simulink model "HVModAL_Fahrzeugmodell"  (R2015b)
settings: Solver=ode1  StartTime=0  StopTime=drp.driving_cycle.tstop  FixedStep=sim_params.Ts  RelTol=1e-5
PreLoadFcn:
  | % Add paths
  | addpath data
  | addpath(genpath('library'))
StartFcn:
  | Simulation.StartTime = tic;
StopFcn:
  | Simulation.DurationTime = toc(Simulation.StartTime);
undefined symbols (not defined in the file or in its folder): Batteries, BMS, BMS_Bat_, C_Nenn_DCDC1, C_Nenn_DCDC2, d2d, DC, DCDC_Converter_efficiency, DcDc_Converters, Dcl, drp, drv, elm, gen, gin, Hdc, hdc, HV, hvb, Hvb, ice, ldc, lib_dcl, lib_hdc, lib_hvb, lib_veh, Link, lossestable, mask_LUT_OCV, mask_LUT_OCV_SOC, mask_LUT_OCV_Temperature, mask_LUT_R, mask_LUT_Rs, mask_LUT_Rs_SOC, mask_LUT_Rs_Temperature, sim_params, speedvec, torquevec, tri, veh, Veh, Vehicle_Chassis
libraries: simulink x29, lib_tri_modules x7, lib_hdc_module x5, lib_gearbox x4, lib_hvb_battery_pack x3, cstblocks x3, PowerLimitBlock x2, MultiCellLibrary x2, lib_aux x1, lib_drv x1, lib_gen x1, lib_elm x1
(part 4 of 7)

== system HVModAL_Fahrzeugmodell/Traction Inverters (Tri)/Tri1/Thermal Model ==
  note: set enable equal 1 for Foster model
      | set enable equal 0 for junction model
  Plosses : Inport
  at_Ambient : Inport  Port=2
  Constant : Constant  Commented=on  Value=0
  Conventional thermal model : Subsystem  Commented=on
  Enable : Constant  Value=0
  Foster Model : Subsystem
  Logical Operator : Logic  Operator=NOT  Inputs=1  AllPortsSameDT=off  OutDataTypeStr=boolean
  Switch : Switch  Criteria=u2 ~= 0  ZeroCross=off
  Thermal Junction Model : Subsystem
  at_Junction_tri_vec : Outport
  wires:
  Foster Model/1(T_junction) -> Switch/1
  Constant/1 -> Conventional thermal model/Enable
  Thermal Junction Model/1(T_junction) -> Switch/3
  at_Ambient/1 -> Thermal Junction Model/2(T_amb), Foster Model/2(T_amb)
  Plosses/1 -> Thermal Junction Model/1(P_loss_vec), Foster Model/1(P_loss_vec)
  Enable/1 -> Logical Operator/1, Switch/2, Foster Model/Enable
  Switch/1 -> at_Junction_tri_vec/1
  Logical Operator/1 -> Thermal Junction Model/Enable

== system HVModAL_Fahrzeugmodell/Traction Inverters (Tri)/Tri1/Thermal Model old ==
  Plosses : Inport
  at_Ambient : Inport  Port=2
  Scope : Scope
  TJunc : Constant  Value=125
  Thermal Junction Model : Subsystem
  at_Junction : Outport
  wires:
  TJunc/1 -> at_Junction/1
  at_Ambient/1 -> Thermal Junction Model/2(T_amb)
  Plosses/1 -> Thermal Junction Model/1(P_loss_vec)
  Thermal Junction Model/1(T_junction) -> Scope/1

== system HVModAL_Fahrzeugmodell/Traction Inverters (Tri)/Tri1/mean_at_junction ==
  at_junction_tri_vec : Inport
  Constant : Constant  Value=12
  Divide : Product  Inputs=*/
  Sum of Elements : Sum  Inputs=+
  at_junction : Outport
  wires:
  at_junction_tri_vec/1 -> Sum of Elements/1
  Sum of Elements/1 -> Divide/1
  Constant/1 -> Divide/2
  Divide/1 -> at_junction/1

== system HVModAL_Fahrzeugmodell/Vehicle_Chassis (Veh)/Driving Data/Calculate Actual Speed ==
  m_red [kg] : Inport
  F_drive [N] : Inport  Port=2
  Integrator : Integrator
  Product : Product  Inputs=/*  SaturateOnIntegerOverflow=on  InputSameDT=on  OutDataTypeStr=Inherit: Same as first input
  v_actual [m/s] : Outport
  a_actual [m/s] : Outport  Port=2
  wires:
  Product/1 -> Integrator/1, a_actual [m/s]/1  "a_actual [m/s²]"
  Integrator/1 -> v_actual [m/s]/1  "v_actual [m/s]"
  m_red [kg]/1 -> Product/1
  F_drive [N]/1 -> Product/2

== system HVModAL_Fahrzeugmodell/Vehicle_Chassis (Veh)/Driving Data/Conversions ==
  v_actual (m/s) : Inport
  Emg_gearbox_vec : Inport  Port=2
  1/r_dyn : Gain  Gain=1/veh.wheel.radius  SaturateOnIntegerOverflow=on  OutDataTypeStr=Inherit: Same as input  ParamDataTypeStr=Inherit: Same as input
  Bus Selector : BusSelector  OutputSignals=BM on/off,gearboxratio_vec
  Demux : Demux
  Divide{,1..3} (4 alike) : Product  Inputs=*/
  Gain : Gain  Gain=veh.topology.boost_clutch
  Gain1 : Gain  Gain=veh.gearbox.gearbox2.ratio*elm.elm2.phys_avail  SaturateOnIntegerOverflow=on  OutDataTypeStr=Inherit: Same as input  ParamDataTypeStr=Inherit: Same as input
  Gain2 : Gain  Gain=veh.gearbox.gearbox1.ratio*elm.elm1.phys_avail  SaturateOnIntegerOverflow=on  OutDataTypeStr=Inherit: Same as input  ParamDataTypeStr=Inherit: Same as input
  Gain3 : Gain  Gain=veh.gearbox.gearbox3.ratio*elm.elm3.phys_avail  SaturateOnIntegerOverflow=on  OutDataTypeStr=Inherit: Same as input  ParamDataTypeStr=Inherit: Same as input
  Gain4 : Gain  Gain=veh.gearbox.gearbox4.ratio*elm.elm4.phys_avail  SaturateOnIntegerOverflow=on  OutDataTypeStr=Inherit: Same as input  ParamDataTypeStr=Inherit: Same as input
  Logical Operator : Logic  Operator=NOT  AllPortsSameDT=off  OutDataTypeStr=boolean
  Logical Operator1 : Logic  Operator=NOT  AllPortsSameDT=off  OutDataTypeStr=boolean
  Logical Operator2 : Logic  Operator=NOT  AllPortsSameDT=off  OutDataTypeStr=boolean
  Mux : Mux
  Product : Product  Inputs=3
  Product1 : Product  Inputs=3
  Switch : Switch  Criteria=u2 > Threshold
  Switch1 : Switch  Criteria=u2 > Threshold
  Terminator : Terminator
  Terminator2 : Terminator
  Terminator3 : Terminator
  const : Constant  Value=0
  const1 : Constant  Value=0
  "m/s -> km/h" : Gain  Gain=3.6  SaturateOnIntegerOverflow=on  OutDataTypeStr=Inherit: Same as input  ParamDataTypeStr=Inherit: Same as input
  "m/s -> rpm" : Gain  Gain=30/(pi*veh.wheel.radius)  SaturateOnIntegerOverflow=on  OutDataTypeStr=Inherit: Same as input  ParamDataTypeStr=Inherit: Same as input
  veh.topology.boost : Constant  Value=veh.topology.boost
  veh.topology.loc_boost : Constant  Value=veh.topology.loc_boost
  veh_n_motor_vec : Outport
  wires:
  Gain4/1 -> Divide/1
  Divide1/1 -> Mux/3
  Mux/1 -> veh_n_motor_vec/1
  "m/s -> km/h"/1 -> Terminator2/1  "v_actual (km/h)"
  1/r_dyn/1 -> Terminator/1  "n_wheels (rad/s)"
  "m/s -> rpm"/1 -> Terminator3/1, Gain2/1, Gain1/1, Gain3/1, Gain4/1  "n_wheels (rpm)"
  Divide3/1 -> Mux/1
  v_actual (m/s)/1 -> "m/s -> rpm"/1, 1/r_dyn/1, "m/s -> km/h"/1
  Emg_gearbox_vec/1 -> Bus Selector/1
  veh.topology.boost/1 -> Gain/1
  veh.topology.loc_boost/1 -> Logical Operator2/1, Product/3
  Bus Selector/1 -> Logical Operator1/1, Logical Operator/1  "<BM on/off>"
  Divide/1 -> Switch/3
  Product/1 -> Switch/2
  const/1 -> Switch/1
  Logical Operator/1 -> Product/1
  Gain/1 -> Product/2, Product1/2
  Product1/1 -> Switch1/2
  const1/1 -> Switch1/1
  Logical Operator1/1 -> Product1/1
  Switch1/1 -> Mux/2
  Divide2/1 -> Switch1/3
  Logical Operator2/1 -> Product1/3
  Switch/1 -> Mux/4
  Bus Selector/2 -> Demux/1  "<gearboxratio_vec>"
  Demux/4 -> Divide/2
  Gain3/1 -> Divide1/1
  Gain1/1 -> Divide2/1
  Demux/3 -> Divide1/2
  Demux/2 -> Divide2/2
  Gain2/1 -> Divide3/1
  Demux/1 -> Divide3/2

== system HVModAL_Fahrzeugmodell/Vehicle_Chassis (Veh)/Driving Forces/Aerodynamic Resistance ==
  v_desired [m/s] : Inport
  0.5*f_drag*A_front : Gain  Gain=veh.drag_coefficient*veh.front_area*0.5  SaturateOnIntegerOverflow=on  OutDataTypeStr=Inherit: Same as input  ParamDataTypeStr=Inherit: Same as input
  Air density : Gain  Gain=drp.airdensity  SaturateOnIntegerOverflow=on  OutDataTypeStr=Inherit: Same as input  ParamDataTypeStr=Inherit: Same as input
  Math Function : Math  Operator=square  SaturateOnIntegerOverflow=on
  F_aero [N] : Outport
  wires:
  0.5*f_drag*A_front/1 -> Air density/1
  v_desired [m/s]/1 -> Math Function/1
  Math Function/1 -> 0.5*f_drag*A_front/1
  Air density/1 -> F_aero [N]/1

== system HVModAL_Fahrzeugmodell/Vehicle_Chassis (Veh)/Driving Forces/Climbing Resistance ==
  gradient : Inport
  m_total * 9.81 : Gain  Gain=veh.totalweight*9.81  SaturateOnIntegerOverflow=on  OutDataTypeStr=Inherit: Same as input  ParamDataTypeStr=Inherit: Same as input
  sin(grad) : Trigonometry
  F_climb [N] : Outport
  wires:
  m_total * 9.81/1 -> F_climb [N]/1
  sin(grad)/1 -> m_total * 9.81/1
  gradient/1 -> sin(grad)/1

== system HVModAL_Fahrzeugmodell/Vehicle_Chassis (Veh)/Driving Forces/Rolling Resistance ==
  v_actual(m/s) : Inport
  gradient : Inport  Port=2
  9.81*m_total*f_roll : Gain  Gain=(veh.totalweight)*9.81*veh.wheel.rolling_resistance  SaturateOnIntegerOverflow=on  OutDataTypeStr=Inherit: Same as input  ParamDataTypeStr=Inherit: Same as input
  Constant : Constant  Value=0
  Product : Product
  Sign : Signum
  Switch : Switch  Threshold=0.1
  cos(grad) : Trigonometry  Operator=cos
  F_roll [N] : Outport
  wires:
  9.81*m_total*f_roll/1 -> Product/1
  gradient/1 -> cos(grad)/1
  cos(grad)/1 -> 9.81*m_total*f_roll/1
  Sign/1 -> Product/2
  Product/1 -> F_roll [N]/1
  v_actual(m/s)/1 -> Switch/1, Switch/2
  Constant/1 -> Switch/3
  Switch/1 -> Sign/1

== system HVModAL_Fahrzeugmodell/Vehicle_Chassis (Veh)/Wheel Model/  ==
  note: Wenn F_H > Fx : 1
  note: Abstand zwischen zwei Profilteilchen
  note: Länge eines Profilteilchens
  "F_x[N] " : Inport
  wheelLoad[N] : Inport  Port=2
  Abs : Abs
  Compare To Zero : simulink/Logic and Bit Operations/Compare To Zero  relop=>=  OutDataTypeStr=boolean
  Constant : Constant  Value=4
  Constant1 : Constant  Value=false
  Data Store Memory : DataStoreMemory  DataStoreName=Slip  ReadBeforeWriteMsg=warning  WriteAfterWriteMsg=warning  WriteAfterReadMsg=warning  InitialValue=false  ShowAdditionalParam=off  OutDataTypeStr=boolean
  Data Store Read : DataStoreRead  DataStoreName=Slip
  Gain : Gain  Gain=2
  Gain1 : Gain  Gain=2
  Gain2 : Gain  Gain=veh.wheel.coefficient_of_friction
  If : If  IfExpression=u1 <= 2000
  If Action Subsystem : Subsystem  TreatAsAtomicUnit=on
  Product : Product  Inputs=*/**///
  Product1 : Product  Inputs=*///
  Product2 : Product  Inputs=3
  Sqrt : Sqrt  SaturateOnIntegerOverflow=on
  Sum : Sum  Inputs=|++
  Sum1 : Sum  Inputs=+-
  Switch : Switch  Criteria=u2 > Threshold
  WheelRadius[m] : Constant  Value=veh.wheel.radius
  circumferentialTireRigidity[N/m] : Constant  Value=veh.wheel.c_t_rigidity
  distanceTireTread[m] : Constant  Value=veh.wheel.tread_distance
  lengthTireTread[m] : Constant  Value=veh.wheel.tread_length
  radialTireRigidity[N/m] : Constant  Value=veh.wheel.r_t_rigidity
  wheelspin : Outport
  Slip? : Outport  Port=2
  wires:
  Sum/1 -> Gain/1, Product/3
  lengthTireTread[m]/1 -> Sum/1
  distanceTireTread[m]/1 -> Sum/2
  "F_x[N] "/1 -> Product/1, Product2/3
  WheelRadius[m]/1 -> Product/2, Product1/2
  radialTireRigidity[N/m]/1 -> Product1/1, Product/4
  circumferentialTireRigidity[N/m]/1 -> Product/5
  wheelLoad[N]/1 -> Product1/3, Gain2/1, Product/6
  Constant/1 -> Product/7, Gain1/1
  Product/1 -> wheelspin/1
  Gain1/1 -> Product1/4
  Product1/1 -> Sqrt/1
  Sqrt/1 -> Product2/1
  Gain/1 -> Product2/2
  Gain2/1 -> Sum1/1
  Product2/1 -> Abs/1
  Abs/1 -> Sum1/2
  Data Store Read/1 -> Switch/2
  Switch/1 -> Slip?/1
  Constant1/1 -> Switch/3
  Compare To Zero/1 -> Switch/1
  Sum1/1 -> If/1, Compare To Zero/1
  If/1 -> If Action Subsystem/Action

== system HVModAL_Fahrzeugmodell/Vehicle_Chassis (Veh)/Wheel Model/F_x_wheelspin[N] ==
  F_wheel [N] : Inport
  angularVelocity [rad/s] : Inport  Port=2
  wheelload : Inport  Port=3
  Discrete Derivative : simulink/Discrete/Discrete Derivative  gainval=1  ICPrevScaledInput=0.0  InputProcessing=Inherited  OutMin=[]  OutMax=[]  OutDataType=fixdt(1, 16)  OutScaling=2^-10  DoSatur=off
  Gain : Gain  Gain=veh.wheel.coefficient_of_friction
  MinMax : MinMax  Inputs=2
  Product : Product  Inputs=*/
  Sum : Sum  Inputs=|+-
  r_dyn : Constant  Value=veh.wheel.radius
  "wheel_inertia " : Gain  Gain=veh.wheel.inertia
  F_x [N/m] : Outport
  wires:
  angularVelocity [rad/s]/1 -> Discrete Derivative/1
  r_dyn/1 -> Product/2
  F_wheel [N]/1 -> Sum/1
  Product/1 -> Sum/2
  Sum/1 -> MinMax/1
  MinMax/1 -> F_x [N/m]/1
  wheelload/1 -> Gain/1
  Gain/1 -> MinMax/2
  Discrete Derivative/1 -> "wheel_inertia "/1
  "wheel_inertia "/1 -> Product/1

== system HVModAL_Fahrzeugmodell/Vehicle_Chassis (Veh)/Wheel Model/Subsystem ==
  v_wheel [m/s] : Inport
  v/r : Gain  Gain=1/veh.wheel.radius
  angularVelocity[rad/s] : Outport
  wires:
  v_wheel [m/s]/1 -> v/r/1
  v/r/1 -> angularVelocity[rad/s]/1

== system HVModAL_Fahrzeugmodell/Vehicle_Chassis (Veh)/Wheel Model/wheelspin ==
  angularVelocity[rad/s] : Inport
  "wheelspin " : Inport  Port=2
  a_actual [m/s^2] : Inport  Port=3
  Slip? : Inport  Port=4
  v_wheel : Inport  Port=5
  Constant : Constant
  Constant1 : Constant
  Product : Product
  Product1 : Product  Inputs=*/
  Product2 : Product
  Sum : Sum  Inputs=|++  SaturateOnIntegerOverflow=on
  Sum1 : Sum  Inputs=|+-
  Switch : Switch  Criteria=u2 > Threshold
  Switch1 : Switch  Criteria=u2 ~= 0
  Switch2 : Switch  Criteria=u2 > Threshold
  rdyn : Constant  Value=veh.wheel.radius
  v_actual [m/s] : Outport
  wires:
  rdyn/1 -> Product/1
  angularVelocity[rad/s]/1 -> Product/2
  a_actual [m/s^2]/1 -> Switch/2
  Constant/1 -> Switch1/3, Sum/2
  Product/1 -> Product1/1, Product2/1
  Product1/1 -> Switch/3
  Sum1/1 -> Product2/2
  Product2/1 -> Switch/1
  Constant1/1 -> Sum1/1
  "wheelspin "/1 -> Sum1/2, Sum/1
  Sum/1 -> Switch1/2, Switch1/1
  Switch1/1 -> Product1/2
  Slip?/1 -> Switch2/2
  Switch/1 -> Switch2/1
  v_wheel/1 -> Switch2/3
  Switch2/1 -> v_actual [m/s]/1

== system HVModAL_Fahrzeugmodell/Visualization (Vis)/Subsystem1/Auxillaries (aux) ==
  Bus Selector : BusSelector  OutputSignals=Aux_P_lv_bat,Aux_P_dcLink
  Aux_P_lv_bat : Outport
  Aux_P_dcLink : Outport  Port=2
  wires:
  [Aux_BusPB_ToLogging] -> Bus Selector/1
  Bus Selector/1 -> Aux_P_lv_bat/1  "<Aux_P_lv_bat>"
  Bus Selector/2 -> Aux_P_dcLink/1  "<Aux_P_dcLink>"

== system HVModAL_Fahrzeugmodell/Visualization (Vis)/Subsystem1/DC-Link (Dcl) ==
  Bus Selector2 : BusSelector  OutputSignals=Dcl_U,Dcl_P_total,Dcl_P_totalwoHdcPdcLink,Hdc_P_dcLink
  Dcl_U : Outport
  Dcl_P_total : Outport  Port=2
  Dcl_P_totalwoHdcPdc : Outport  Port=3
  Hdc_P_dcLink : Outport  Port=4
  wires:
  [Dcl_BusPB_toworkspace] -> Bus Selector2/1
  Bus Selector2/1 -> Dcl_U/1  "<Dcl_U>"
  Bus Selector2/2 -> Dcl_P_total/1  "<Dcl_P_total>"
  Bus Selector2/3 -> Dcl_P_totalwoHdcPdc/1  "<Dcl_P_totalwoHdcPdcLink>"
  Bus Selector2/4 -> Hdc_P_dcLink/1  "<Hdc_P_dcLink>"

== system HVModAL_Fahrzeugmodell/Visualization (Vis)/Subsystem1/DC//DC Converter (hdc) ==
  Bus Selector : BusSelector  OutputSignals=Hdc_P_bat_vec,Hdc_P_dcLink_vec,Hdc_fac_eta_vec,Hdc_P_losses_vec
  Bus Selector1 : BusSelector  OutputSignals=Hdc_flg_error_vec,Hdc_P_max_vec,Hdc_at_Junction_vec
  Hdc_P_bat_vec : Outport
  Hdc_P_dclink_vec : Outport  Port=2
  Hdc_P_losses_vec : Outport  Port=3
  Hdc_fac_eta_vec : Outport  Port=4
  Hdc_error_vec : Outport  Port=5
  Hdc_Pmax_vec : Outport  Port=6
  Hdc_at_Junction_vec : Outport  Port=7
  wires:
  [Hdc_PBBus_toWorkspace] -> Bus Selector/1
  [Hdc_SWBus_toWorkspace] -> Bus Selector1/1
  Bus Selector/1 -> Hdc_P_bat_vec/1  "<Hdc_P_bat_vec>"
  Bus Selector/2 -> Hdc_P_dclink_vec/1  "<Hdc_P_dcLink_vec>"
  Bus Selector/3 -> Hdc_fac_eta_vec/1  "<Hdc_fac_eta_vec>"
  Bus Selector/4 -> Hdc_P_losses_vec/1  "<Hdc_P_losses_vec>"
  Bus Selector1/1 -> Hdc_error_vec/1  "<Hdc_flg_error_vec>"
  Bus Selector1/3 -> Hdc_at_Junction_vec/1  "<Hdc_at_Junction_vec>"
  Bus Selector1/2 -> Hdc_Pmax_vec/1  "<Hdc_P_max_vec>"

== system HVModAL_Fahrzeugmodell/Visualization (Vis)/Subsystem1/Driver (Drv) ==
  Bus Selector : BusSelector  OutputSignals=Drv_fac_PedAc
  Bus Selector1 : BusSelector  OutputSignals=Emg_T_elDemand_vec,Emg_T_mechDemand
  Bus Selector2 : BusSelector  OutputSignals=Drp_v_vehDesired
  Gain1 : Gain  Gain=3.6
  Sum of Elements : Sum  Inputs=+
  fac_pedAcc : Outport
  Emg_T_el_demand : Outport  Port=2
  Emg_T_mech_demand : Outport  Port=3
  v_cycle(km/h) : Outport  Port=4
  wires:
  Bus Selector/1 -> fac_pedAcc/1  "<Drv_fac_PedAc>"
  [Drv_SWBus_toworkspace] -> Bus Selector/1
  [EMG_BusSW_ToLogging] -> Bus Selector1/1
  Bus Selector1/2 -> Emg_T_mech_demand/1  "<Emg_T_mechDemand>"
  Bus Selector1/1 -> Sum of Elements/1  "<Emg_T_elDemand_vec>"
  Sum of Elements/1 -> Emg_T_el_demand/1
  Gain1/1 -> v_cycle(km/h)/1  "v_cycle(km/h)"
  [Drp_SWBus_toworkspace] -> Bus Selector2/1
  Bus Selector2/1 -> Gain1/1  "<Drp_v_vehDesired>"

== system HVModAL_Fahrzeugmodell/Visualization (Vis)/Subsystem1/EMS ==
  Bus Selector : BusSelector  OutputSignals=Emg_fac_powerDistribution_vec,Emg_T_elDemand_vec,Emg_Degradation_vec
  Demux : Demux  Commented=on  Outputs=5
  Demux1 : Demux
  Emg_fac_powerDristri_Bat1 : Outport
  Emg_fac_powerDristri_Bat2 : Outport  Port=2
  Emg_fac_powerDristri_Bat3 : Outport  Port=3
  Emg_fac_powerDristri_Bat4 : Outport  Port=4
  Emg_fac_powerDristri_Bat5 : Outport  Port=5
  Emg_T_elDemand_Inv1 : Outport  Port=6
  Emg_T_elDemand_Inv2 : Outport  Port=7
  Emg_Degradation : Outport  Port=8
  wires:
  Demux/1 -> Emg_fac_powerDristri_Bat1/1
  Demux/2 -> Emg_fac_powerDristri_Bat2/1
  Demux/3 -> Emg_fac_powerDristri_Bat3/1
  Demux/4 -> Emg_fac_powerDristri_Bat4/1
  Demux/5 -> Emg_fac_powerDristri_Bat5/1
  Demux1/1 -> Emg_T_elDemand_Inv1/1
  Demux1/2 -> Emg_T_elDemand_Inv2/1
  [EMG_BusSW_ToLogging] -> Bus Selector/1
  Bus Selector/1 -> Demux/1  "<Emg_fac_powerDistribution_vec>"
  Bus Selector/2 -> Demux1/1  "<Emg_T_elDemand_vec>"
  Bus Selector/3 -> Emg_Degradation/1  "<Emg_Degradation_vec>"

== system HVModAL_Fahrzeugmodell/Visualization (Vis)/Subsystem1/Elm ==
  Bus Selector : BusSelector  OutputSignals=Elm_T_el_vec,Elm_I_abc_vec,Elm_P_TD_actual_vec
  Bus Selector1 : BusSelector  OutputSignals=Elm_P_losses_vec,Tri_Pmax_elm_vec,elm_at_endWindingsMagnet_vec
  Demux : Demux
  Elm_T_el_vec : Outport
  Elm_P_actual_vec : Outport  Port=2
  Elm_P_losses_vec : Outport  Port=3
  Elm1_I_abc : Outport  Port=4
  Elm_Pmax_vec : Outport  Port=5
  Elm_at_endWindingsMagnet_vec : Outport  Port=6
  wires:
  [Elm_BusPB_toworkspace] -> Bus Selector/1
  Bus Selector/1 -> Elm_T_el_vec/1  "<Elm_T_el_vec>"
  Bus Selector/2 -> Demux/1  "<Elm_I_abc_vec>"
  Demux/1 -> Elm1_I_abc/1  "Elm_I_abc"
  Bus Selector/3 -> Elm_P_actual_vec/1  "<Elm_P_TD_actual_vec>"
  [Tri_BusSW_toWorkspace] -> Bus Selector1/1
  Bus Selector1/1 -> Elm_P_losses_vec/1  "<Elm_P_losses_vec>"
  Bus Selector1/2 -> Elm_Pmax_vec/1  "<Tri_Pmax_elm_vec>"
  Bus Selector1/3 -> Elm_at_endWindingsMagnet_vec/1  "<elm_at_endWindingsMagnet_vec>"

== system HVModAL_Fahrzeugmodell/Visualization (Vis)/Subsystem1/HV-Batteries (hvb) ==
  Abs : Abs
  Add : Sum
  Bus Selector : BusSelector  OutputSignals=PB_Bat1,PB_Bat2
  Bus Selector1 : BusSelector  OutputSignals=Total_Voltage_V,Total_Current_A,SOC_Vector_Percent,Total_Dissipation_Power_W
  Bus Selector2 : BusSelector  OutputSignals=Total_Voltage_V,Total_Current_A,SOC_Vector_Percent
  Bus Selector3 : BusSelector  OutputSignals=SB_Bat1,SB_Bat2
  Bus Selector4 : BusSelector  OutputSignals=P_max_discharge_10s_W
  Bus Selector5 : BusSelector  OutputSignals=P_max_discharge_10s_W
  Constant : Constant  Value=0
  Display : Display
  Display1 : Display
  Display2 : Display
  Gain : Gain  Gain=1/3600
  Gain1 : Gain  Gain=1/3600
  Gain2 : Gain  Gain=1/3600
  Integrator : Integrator
  Integrator1 : Integrator
  Integrator2 : Integrator
  Product : Product
  Product1 : Product
  Switch : Switch  Criteria=u2 > Threshold
  Switch1 : Switch  Criteria=u2 > Threshold
  Hvb_Bat1_U : Outport
  Hvb_Bat1_I : Outport  Port=2
  Hvb_Bat1_P : Outport  Port=3
  Hvb_Bat1_SOC : Outport  Port=4
  Hvb_Bat2_U : Outport  Port=5
  Hvb_Bat2_I : Outport  Port=6
  Hvb_Bat2_P : Outport  Port=7
  Hvb_Bat2_SOC : Outport  Port=8
  Hvb_Bat1_P_max_disch : Outport  Port=9
  Hvb_Bat2_P_max_disch : Outport  Port=10
  Hvb_Bat_P_max_disch : Outport  Port=11
  Hvb_Bat1_Plosses : Outport  Port=12
  wires:
  [Hvb_PBbus_toworkspace] -> Bus Selector/1
  Bus Selector/1 -> Bus Selector1/1  "<PB_Bat1>"
  Bus Selector/2 -> Bus Selector2/1  "<PB_Bat2>"
  Bus Selector1/1 -> Product/1, Hvb_Bat1_U/1  "<Total_Voltage_V>"
  Bus Selector1/2 -> Product/2, Hvb_Bat1_I/1  "<Total_Current_A>"
  Bus Selector1/3 -> Hvb_Bat1_SOC/1  "<SOC_Vector_Percent>"
  Product/1 -> Switch/1, Switch1/3, Switch1/2, Switch/2, Abs/1, Hvb_Bat1_P/1  "Hvb_Bat1_P"
  Bus Selector2/1 -> Hvb_Bat2_U/1, Product1/1  "<Total_Voltage_V>"
  Bus Selector2/2 -> Product1/2, Hvb_Bat2_I/1  "<Total_Current_A>"
  Bus Selector2/3 -> Hvb_Bat2_SOC/1  "<SOC_Vector_Percent>"
  Product1/1 -> Hvb_Bat2_P/1  "Hvb_Bat2_P"
  [Hvb_SWbus_toworkspace] -> Bus Selector3/1
  Bus Selector3/1 -> Bus Selector4/1  "<SB_Bat1>"
  Bus Selector3/2 -> Bus Selector5/1  "<SB_Bat2>"
  Bus Selector4/1 -> Add/1, Hvb_Bat1_P_max_disch/1  "<P_max_discharge_10s_W>"
  Bus Selector5/1 -> Add/2, Hvb_Bat2_P_max_disch/1  "<P_max_discharge_10s_W>"
  Add/1 -> Hvb_Bat_P_max_disch/1
  Bus Selector1/4 -> Hvb_Bat1_Plosses/1  "<Total_Dissipation_Power_W>"
  Switch/1 -> Integrator/1
  Constant/1 -> Switch1/1, Switch/3
  Switch1/1 -> Integrator1/1
  Abs/1 -> Integrator2/1
  Integrator1/1 -> Gain1/1
  Integrator/1 -> Gain/1
  Integrator2/1 -> Gain2/1
  Gain2/1 -> Display/1
  Gain/1 -> Display2/1
  Gain1/1 -> Display1/1

== system HVModAL_Fahrzeugmodell/Visualization (Vis)/Subsystem1/LV-DCDC (ldc) ==
  Bus Selector1 : BusSelector  OutputSignals=Ldc_Pmax_vec,Ldc_atJunction_vec,Ldc_error_vec
  Bus Selector2 : BusSelector  OutputSignals=Ldc_P_LvBat,Ldc_P_HvBat_vec,Ldc_P_dcLink
  Ldc_P_Lv_bat : Outport
  Ldc_P_HvBat_vec : Outport  Port=2
  Ldc_P_dcLink : Outport  Port=3
  Ldc_atJunction_vec : Outport  Port=4
  Ldc_Pmax_vec : Outport  Port=5
  Ldc_error_vec : Outport  Port=6
  wires:
  [LDC_BusSB_ToLogging] -> Bus Selector1/1
  Bus Selector1/1 -> Ldc_Pmax_vec/1  "<Ldc_Pmax_vec>"
  Bus Selector1/2 -> Ldc_atJunction_vec/1  "<Ldc_atJunction_vec>"
  Bus Selector1/3 -> Ldc_error_vec/1  "<Ldc_error_vec>"
  [LDC_BusPB_ToLogging] -> Bus Selector2/1
  Bus Selector2/1 -> Ldc_P_Lv_bat/1  "<Ldc_P_LvBat>"
  Bus Selector2/2 -> Ldc_P_HvBat_vec/1  "<Ldc_P_HvBat_vec>"
  Bus Selector2/3 -> Ldc_P_dcLink/1  "<Ldc_P_dcLink>"

== system HVModAL_Fahrzeugmodell/Visualization (Vis)/Subsystem1/Subsystem1 ==
  Bus Selector1 : BusSelector  OutputSignals=Drp_v_vehDesired
  Bus Selector2 : BusSelector  OutputSignals=Veh_random
  Gain : Gain  Gain=3.6
  Gain1 : Gain  Gain=3.6
  Sum : Sum  Inputs=+-
  v_deviation(km/h) : Outport
  wires:
  Bus Selector1/1 -> Gain1/1  "<Drp_v_vehDesired>"
  Sum/1 -> v_deviation(km/h)/1  "v_deviation(km/h)"
  Gain/1 -> Sum/2  "v_actual(km/h)"
  [Drp_SWBus_toworkspace] -> Bus Selector1/1
  Bus Selector2/1 -> Gain/1  "<Veh_random>"
  [Veh_SWBus_toworkspace] -> Bus Selector2/1
  Gain1/1 -> Sum/1  "v_cycle(km/h)"

== system HVModAL_Fahrzeugmodell/Visualization (Vis)/Subsystem1/Traction Inverters(Tri) ==
  Bus Selector1 : BusSelector  OutputSignals=Tri_Pmax_vec,Tri_fac_eta,Tri_at_Junction_vec
  Bus Selector2 : BusSelector  OutputSignals=Tri_P_dcLink_vec,Tri_P_losses_vec
  Tri_P_dcLink : Outport
  Tri_P_losses : Outport  Port=2
  Tri_eta : Outport  Port=3
  Tri_Pmax : Outport  Port=4
  Tri_atJunction : Outport  Port=5
  wires:
  [Tri_BusPB_toWorkspace] -> Bus Selector2/1
  [Tri_BusSW_toWorkspace] -> Bus Selector1/1
  Bus Selector2/1 -> Tri_P_dcLink/1  "<Tri_P_dcLink_vec>"
  Bus Selector2/2 -> Tri_P_losses/1  "<Tri_P_losses_vec>"
  Bus Selector1/1 -> Tri_Pmax/1  "<Tri_Pmax_vec>"
  Bus Selector1/2 -> Tri_eta/1  "<Tri_fac_eta>"
  Bus Selector1/3 -> Tri_atJunction/1  "<Tri_at_Junction_vec>"

== system HVModAL_Fahrzeugmodell/Visualization (Vis)/Subsystem1/Vehicle (veh) ==
  Bus Selector2 : BusSelector  OutputSignals=Veh_DrivingForces_N,Veh_a_actual,Veh_random,Veh_v_actual,Veh_Ploss_gearbox_vec
  Demux : Demux  Outputs=5
  Sum : Sum  Inputs=+-|
  Sum of Elements : Sum  Inputs=+
  Veh_F_aero : Outport
  Veh_F_climb : Outport  Port=2
  Veh_F_drive : Outport  Port=3
  Veh_F_roll : Outport  Port=4
  Veh_F_acc : Outport  Port=5
  Veh_a_actual : Outport  Port=6
  Veh_v_actual : Outport  Port=7
  Veh_v_actual-v_wheel : Outport  Port=8
  Veh_Ploss_gearbox : Outport  Port=9
  wires:
  [Veh_SWBus_toworkspace] -> Bus Selector2/1
  Bus Selector2/1 -> Demux/1  "<Veh_DrivingForces_N>"
  Demux/1 -> Veh_F_acc/1
  Demux/2 -> Veh_F_aero/1
  Demux/3 -> Veh_F_climb/1
  Demux/4 -> Veh_F_drive/1
  Demux/5 -> Veh_F_roll/1
  Bus Selector2/2 -> Veh_a_actual/1  "<Veh_a_actual>"
  Bus Selector2/3 -> Sum/1, Veh_v_actual/1  "<Veh_random>"
  Bus Selector2/4 -> Sum/2  "<Veh_v_actual>"
  Sum/1 -> Veh_v_actual-v_wheel/1
  Bus Selector2/5 -> Sum of Elements/1  "<Veh_Ploss_gearbox_vec>"
  Sum of Elements/1 -> Veh_Ploss_gearbox/1

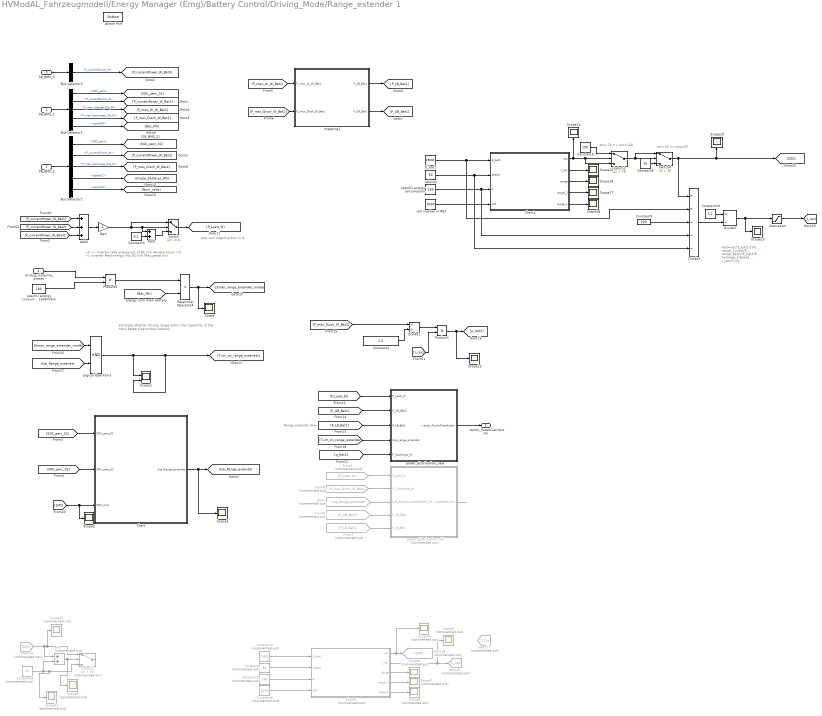
== system HVModAL_Fahrzeugmodell/Energy Manager (Emg)/Battery Control/Driving_Mode/Range_extender 1 ==
  note: pos. and negative
      | but != 0
  note: >0 --> Inverter take energy out of DC link (Acceleration)
      | <0 --> Inverter feed energy into DC link (Recuperation)
  note: Range extender 5kw
  note: estimate whether driving range within the capability of the main battery(secondary battery
  note: soc<30 => soc=30
  note: soc>79 => soc=100
  note: rest=soc*E_bat1/100;...
      |  range_1=rest/E;...
      | range_bat1=E_bat1/E;...
      |  t=range_1/speed;...
      |  I_rex=3.1/t;...
  SB_BMS_1 : Inport
  SB_BMS_2 : Inport  Port=2
  SB_BMS_3 : Inport  Port=3
  driving_distance_preset : Inport  Port=4
  Action Port : ActionPort
  Add : Sum  Commented=on
  Add1 : Sum
  Add2 : Sum  Inputs=+++
  Bus Selector1 : BusSelector  OutputSignals=SOC_perc,P_currentPower_W,P_max_charge_10s_W,P_max_discharge_10s_W,signal20
  Bus Selector2 : BusSelector  OutputSignals=SOC_perc,P_currentPower_W,P_max_discharge_10s_W,signal21,signal22
  Bus Selector3 : BusSelector  OutputSignals=P_currentPower_W
  Chart : Stateflow chart  TreatAsAtomicUnit=on
      settings: PermitHierarchicalResolution=ParametersOnly
  Chart1 : Stateflow chart  TreatAsAtomicUnit=on
      settings: PermitHierarchicalResolution=ParametersOnly
  Chart3 : Stateflow chart  Commented=on  TreatAsAtomicUnit=on
      settings: PermitHierarchicalResolution=ParametersOnly
  Constant : Constant  Commented=on  Value=50
  Constant1 : Constant  Commented=on  Value=25000
  Constant10 : Constant  Value=3.1
  Constant2 : Constant  Value=2.5
  Constant3 : Constant  Value=0.1
  Constant4 : Constant  Commented=on  Value=10
  Constant5 : Constant  Value=100
  Constant6 : Constant  Commented=on  Value=4200
  Constant7 : Constant  Commented=on  Value=160
  Constant8 : Constant  Value=30
  Constant9 : Constant  Value=100
  Divide1 : Product  Inputs=*/
  Divide2 : Product  Inputs=**///
  Divide3 : Product  Inputs=*/
  E_bat1 : Constant  Value=25000
  From : From  Commented=on  GotoTag=Use_Range_extender  TagVisibility=global
  From1 : From  Commented=on  GotoTag=P_Load_W
  From10 : From  Commented=on  GotoTag=SOC
  From7 : From  Commented=on  GotoTag=P_LB_Bat1
  From8 : From  Commented=on  GotoTag=P_UB_Bat1
  From9 : From  Commented=on  GotoTag=P_max_Disch_W_Bat2
  Gain : Gain  Gain=-1
  Goto17 : Goto  Commented=on  GotoTag=I_rex
  Goto18 : Goto  Commented=on  GotoTag=SOC
  Goto21 : Goto  Commented=on  GotoTag=I_rex
  Logical Operator3 : Logic  AllPortsSameDT=off  OutDataTypeStr=boolean
  Product1 : Product
  Product2 : Product
  Relational Operator4 : RelationalOperator  Operator=>  OutDataTypeStr=boolean
  Saturation : Saturate  UpperLimit=3  LowerLimit=0
  Scope{,2..3,12..19} (11 alike) : Scope
  Scope1 : Scope  NumInputPorts=2
  Scope{4..11} (8 alike) : Scope  Commented=on
  Switch : Switch  Criteria=u2 ~= 0  Threshold=0.5
  Switch1 : Switch  Commented=on  Criteria=u2 > Threshold  Threshold=20
  Switch2 : Switch  Criteria=u2 > Threshold  Threshold=79
  Switch4 : Switch  Criteria=u2 > Threshold  Threshold=30
  cell number in REX : Constant  Value=4000
  mapping1 : Subsystem  AncestorBlock=PowerDistribution_Dynamic_algo/Dynamic_power_distribution_1av_HE_AND_2av_HP/mapping1  TreatAsAtomicUnit=on
  power_distribution_new : Subsystem
  power_distribution_old : Subsystem  Commented=on
  specific energy consumption : Constant  Value=160
  specific energy consumption 160Wh/Km : Constant  Value=160
  velocity : Constant  Value=50
  vector_PowerDistribution : Outport
  tag scope: Use_Range_extender=global
  wires:
  Chart/1(Use_Range_extender) -> Scope3/1, [Use_Range_extender]
  Gain/1 -> Add1/1, Switch/2, Switch/1
  Constant3/1 -> Add1/2
  Add1/1 -> Switch/3
  [P_currentPower_W_Bat2] -> Add2/2
  [P_currentPower_W_Bat1] -> Add2/1
  Add2/1 -> Gain/1
  SB_BMS_1/1 -> Bus Selector1/1
  SB_BMS_2/1 -> Bus Selector2/1
  [SOC_perc_02] -> Chart/2(SOC_perc_02)
  [SOC_perc_01] -> Chart/1(SOC_perc_01)
  Bus Selector2/1 -> [SOC_perc_02]  "<SOC_perc>"
  Bus Selector2/2 -> [P_currentPower_W_Bat2]  "<P_currentPower_W>"
  Bus Selector1/2 -> [P_currentPower_W_Bat1]  "<P_currentPower_W>"
  Bus Selector1/1 -> [SOC_perc_01]  "<SOC_perc>"
  SB_BMS_3/1 -> Bus Selector3/1
  Bus Selector3/1 -> [P_currentPower_W_Bat3]  "<P_currentPower_W>"
  [P_currentPower_W_Bat3] -> Add2/3
  From1/1 -> power_distribution_old/1(P_Load_W)
  From9/1 -> power_distribution_old/2(P2_discharge_W)
  From/1 -> power_distribution_old/3(Use_Range_extender)
  Bus Selector1/3 -> [P_max_ch_W_Bat1]  "<P_max_charge_10s_W>"
  Bus Selector1/4 -> [P_max_Disch_W_Bat1]  "<P_max_discharge_10s_W>"
  [P_max_ch_W_Bat1] -> mapping1/1(P_max_ch_W_Bat1)
  [P_max_Disch_W_Bat1] -> mapping1/2(P_max_Disch_W_Bat1)
  mapping1/1(P_LB_Bat1) -> [P_LB_Bat1]
  mapping1/2(P_UB_Bat1) -> [P_UB_Bat1]
  From8/1 -> power_distribution_old/4(P_UB_Bat1)
  From7/1 -> power_distribution_old/5(P_LB_Bat1)
  Bus Selector2/3 -> [P_max_Disch_W_Bat2]  "<P_max_discharge_10s_W>"
  Switch/1 -> [P_Load_W]
  power_distribution_old/1(vector_PowerDistribution) -> ?
  Bus Selector1/5 -> [Bat_Wh]  "<signal20>"
  [Bat_Wh] -> Relational Operator4/2
  [P_Load_W] -> power_distribution_new/1(P_Load_W)
  [p_bat2] -> power_distribution_new/5(P_discharge_W)
  [P_LB_Bat1] -> power_distribution_new/3(P_LB_Bat1)
  [P_UB_Bat1] -> power_distribution_new/2(P_UB_Bat1)
  power_distribution_new/1(vector_PowerDistribution) -> vector_PowerDistribution/1
  Relational Operator4/1 -> Scope/1, [Enter_range_extender_mode]
  [Enter_range_extender_mode] -> Logical Operator3/1
  [Use_Range_extender] -> Logical Operator3/2
  [Turn_on_range_extender] -> power_distribution_new/4(Use_range_extender)
  Logical Operator3/1 -> Scope1/2, [Turn_on_range_extender], Scope1/1
  Product1/1 -> Scope12/1, [p_bat2]
  Constant2/1 -> Divide1/2
  [P_max_Disch_W_Bat2] -> Divide1/1
  Divide1/1 -> Product1/1
  Bus Selector2/4 -> [Single_battery2_Wh]  "<signal21>"
  Bus Selector2/5 -> [Num_cells]  "<signal22>"
  Constant/1 -> Chart3/2(speed)
  Constant7/1 -> Chart3/3(E)
  Chart3/2(I_rex) -> Goto21/1, Scope5/1
  Chart3/3(range) -> Scope6/1
  Chart3/1(soc) -> Goto18/1, Scope4/1
  Chart3/4(range_2) -> Scope7/1
  Chart3/5(range_1) -> Scope8/1
  From10/1 -> Add/1, Scope10/1, Switch1/1
  Constant4/1 -> Add/2, Scope11/1, Switch1/3
  Add/1 -> Scope9/1, Switch1/2
  [SOC] -> Chart/3(SOC_limit), Scope2/1
  Constant6/1 -> Chart3/4(cell)
  Constant1/1 -> Chart3/1(E_bat1)
  driving_distance_preset/1 -> Product2/1
  specific energy consumption 160Wh/Km/1 -> Product2/2
  Product2/1 -> Relational Operator4/1
  [I_rex] -> Product1/2
  Constant5/1 -> Switch2/1
  Switch2/1 -> Switch4/1, Switch4/2
  Constant8/1 -> Switch4/3
  Divide2/1 -> Divide3/2
  Switch4/1 -> [SOC], Scope19/1, Divide2/1
  Constant9/1 -> Divide2/3
  Divide3/1 -> Saturation/1, Scope13/1
  Constant10/1 -> Divide3/1
  velocity/1 -> Divide2/5, Chart1/2(speed)
  specific energy consumption/1 -> Divide2/4, Chart1/3(E)
  Chart1/2(I_rex) -> Scope15/1
  Chart1/1(soc) -> Scope14/1, Switch2/3, Switch2/2
  Chart1/3(range) -> Scope16/1
  Chart1/4(range_2) -> Scope17/1
  Chart1/5(range_1) -> Scope18/1
  cell number in REX/1 -> Chart1/4(cell)
  E_bat1/1 -> Divide2/2, Chart1/1(E_bat1)
  Saturation/1 -> [I_rex]

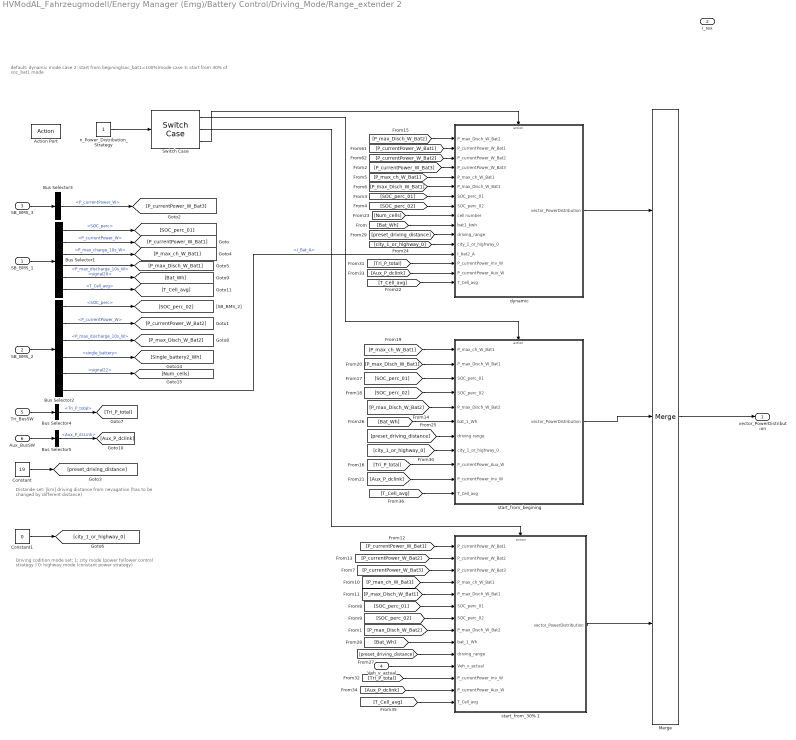
== system HVModAL_Fahrzeugmodell/Energy Manager (Emg)/Battery Control/Driving_Mode/Range_extender 2 ==
  note: default: dynamic mode
      | case 2: start from begining(soc_bat1=100%)mode
      | case 3: start from 30% of soc_bat1 mode
  note: Distande set: [km]
      | driving distance from nevagation
      | (has to be changed by different distance)
  note: Driving codition mode set:
      | 1: city mode (power follower control strategy )
      | 0: highway mode (constant power strategy)
  SB_BMS_1 : Inport
  SB_BMS_2 : Inport  Port=2
  SB_BMS_3 : Inport  Port=3
  Veh_v_actual : Inport  Port=4
  Tri_BusSW : Inport  Port=5
  "Aux_BusSW " : Inport  Port=6
  Action Port : ActionPort  ActionType=case
  Bus Selector1 : BusSelector  OutputSignals=SOC_perc,P_currentPower_W,P_max_charge_10s_W,P_max_discharge_10s_W,signal20,T_Cell_avg
  Bus Selector2 : BusSelector  OutputSignals=SOC_perc,P_currentPower_W,P_max_discharge_10s_W,single_battery,signal22,I_Bat_A
  Bus Selector3 : BusSelector  OutputSignals=P_currentPower_W
  Bus Selector4 : BusSelector  OutputSignals=Tri_P_total
  Bus Selector5 : BusSelector  OutputSignals=Aux_P_dcLink
  Constant : Constant  Value=19
  Constant1 : Constant  Value=0
  Merge : Merge  Inputs=3
  Switch Case : SwitchCase  CaseConditions={2, 3}
  dynamic : Subsystem
  n_Power_Distribution_Strategy : Constant
  start_from_30% 1 : Subsystem
  "start_from_begining " : Subsystem
  vector_PowerDistribution : Outport
  I_rex : Outport  Port=2
  wires:
  SB_BMS_1/1 -> Bus Selector1/1
  SB_BMS_2/1 -> Bus Selector2/1
  Bus Selector2/1 -> [SOC_perc_02]  "<SOC_perc>"
  Bus Selector2/2 -> [P_currentPower_W_Bat2]  "<P_currentPower_W>"
  Bus Selector1/2 -> [P_currentPower_W_Bat1]  "<P_currentPower_W>"
  Bus Selector1/1 -> [SOC_perc_01]  "<SOC_perc>"
  SB_BMS_3/1 -> Bus Selector3/1
  Bus Selector3/1 -> [P_currentPower_W_Bat3]  "<P_currentPower_W>"
  Bus Selector1/3 -> [P_max_ch_W_Bat1]  "<P_max_charge_10s_W>"
  Bus Selector1/4 -> [P_max_Disch_W_Bat1]  "<P_max_discharge_10s_W>"
  Bus Selector2/3 -> [P_max_Disch_W_Bat2]  "<P_max_discharge_10s_W>"
  Bus Selector1/5 -> [Bat_Wh]  "<signal20>"
  Bus Selector2/4 -> [Single_battery2_Wh]  "<single_battery>"
  Bus Selector2/5 -> [Num_cells]  "<signal22>"
  [P_max_Disch_W_Bat2] -> dynamic/1(P_max_Disch_W_Bat2)
  [P_currentPower_W_Bat1] -> dynamic/2(P_currentPower_W_Bat1)
  [P_currentPower_W_Bat2] -> dynamic/3(P_currentPower_W_Bat2)
  [P_currentPower_W_Bat3] -> dynamic/4(P_currentPower_W_Bat3)
  [P_max_ch_W_Bat1] -> dynamic/5(P_max_ch_W_Bat1)
  [P_max_Disch_W_Bat1] -> dynamic/6(P_max_Disch_W_Bat1)
  [SOC_perc_01] -> dynamic/7(SOC_perc_01)
  [SOC_perc_02] -> dynamic/8(SOC_perc_02)
  n_Power_Distribution_Strategy/1 -> Switch Case/1
  start_from_30% 1/1(vector_PowerDistribution) -> Merge/3
  [P_max_Disch_W_Bat2] -> "start_from_begining "/5(P_max_Disch_W_Bat2)
  [P_max_ch_W_Bat1] -> "start_from_begining "/1(P_max_ch_W_Bat1)
  [P_max_Disch_W_Bat1] -> "start_from_begining "/2(P_max_Disch_W_Bat1)
  [SOC_perc_01] -> "start_from_begining "/3(SOC_perc_01)
  [SOC_perc_02] -> "start_from_begining "/4(SOC_perc_02)
  Switch Case/3 -> dynamic/Action
  Switch Case/2 -> start_from_30% 1/Action
  Switch Case/1 -> "start_from_begining "/Action
  Merge/1 -> vector_PowerDistribution/1
  dynamic/1(vector_PowerDistribution) -> Merge/1
  Constant/1 -> [preset_driving_distance]
  [Bat_Wh] -> dynamic/10(bat1_kwh)
  [Num_cells] -> dynamic/9(cell number)
  [preset_driving_distance] -> dynamic/11(driving_range)
  [preset_driving_distance] -> "start_from_begining "/7(driving range)
  [Bat_Wh] -> "start_from_begining "/6(bat_1_Wh)
  [P_currentPower_W_Bat1] -> start_from_30% 1/1(P_currentPower_W_Bat1)
  [P_currentPower_W_Bat2] -> start_from_30% 1/2(P_currentPower_W_Bat2)
  [P_currentPower_W_Bat3] -> start_from_30% 1/3(P_currentPower_W_Bat3)
  [P_max_ch_W_Bat1] -> start_from_30% 1/4(P_max_ch_W_Bat1)
  [P_max_Disch_W_Bat1] -> start_from_30% 1/5(P_max_Disch_W_Bat1)
  [SOC_perc_01] -> start_from_30% 1/6(SOC_perc_01)
  [SOC_perc_02] -> start_from_30% 1/7(SOC_perc_02)
  [P_max_Disch_W_Bat2] -> start_from_30% 1/8(P_max_Disch_W_Bat2)
  [preset_driving_distance] -> start_from_30% 1/10(driving_range)
  [Bat_Wh] -> start_from_30% 1/9(bat_1_Wh)
  Constant1/1 -> [city_1_or_highway_0]
  "start_from_begining "/1(vector_PowerDistribution) -> Merge/2
  [city_1_or_highway_0] -> dynamic/12(city_1_or_highway_0)
  [city_1_or_highway_0] -> "start_from_begining "/8(" city_1_or_highway_0")
  Veh_v_actual/1 -> start_from_30% 1/11(Veh_v_actual)
  ? -> I_rex/1
  Bus Selector2/6 -> dynamic/13(I_bat2_A)  "<I_Bat_A>"
  Tri_BusSW/1 -> Bus Selector4/1
  "Aux_BusSW "/1 -> Bus Selector5/1
  Bus Selector4/1 -> [Tri_P_total]  "<Tri_P_total>"
  Bus Selector5/1 -> [Aux_P_dclink]  "<Aux_P_dcLink>"
  [Tri_P_total] -> dynamic/14(P_currentPower_Inv_W)
  [Aux_P_dclink] -> dynamic/15(P_currentPower_Aux_W)
  [Tri_P_total] -> start_from_30% 1/12(P_currentPower_Inv_W)
  [Aux_P_dclink] -> start_from_30% 1/13(P_currentPower_Aux_W)
  [Tri_P_total] -> "start_from_begining "/9(P_currentPower_Aux_W)
  [Aux_P_dclink] -> "start_from_begining "/10(P_currentPower_Inv_W)
  Bus Selector1/6 -> [T_Cell_avg]  "<T_Cell_avg>"
  [T_Cell_avg] -> dynamic/16(T_Cell_avg)
  [T_Cell_avg] -> "start_from_begining "/11(T_Cell_avg)
  [T_Cell_avg] -> start_from_30% 1/14(T_Cell_avg)

== system HVModAL_Fahrzeugmodell/Energy Manager (Emg)/Battery Control/Driving_Mode/Strategy_Maximiziation_Available_Batterypower ==
  note: Maximierung der Leistung
      | - Bei gleichartigen Batterien: Ausgleich des Ladezustands, so dass EOD-Zeitpunkt gleichzeitig erreicht
      | - Bei Einsatz eines HP-Packs
      | 	abhängig von Größe dieses als Boost-Einheit für Lastspitzen nutzen
      | 	Anschließend Nachladen aus HE-Pack (bidirektionale Wandler notwendig)
  SB_BMS_1 : Inport
  SB_BMS_2 : Inport  Port=2
  SB_BMS_3 : Inport  Port=3
  Action Port : ActionPort  ActionType=default
  Bus Selector : BusSelector  OutputSignals=b_Bat_available_b,n_bat_type_ID_i
  Bus Selector1 : BusSelector  OutputSignals=b_Bat_available_b,n_bat_type_ID_i
  Bus Selector2 : BusSelector  OutputSignals=b_Bat_available_b,n_bat_type_ID_i
  Choice_Algorithm : Subsystem
  Constant : Constant
  Dynamic_power_distribution : PowerDistribution_Dynamic/Dynamic_power_distribution
  Logical Operator1 : Logic  AllPortsSameDT=off  OutDataTypeStr=boolean
  Logical Operator2 : Logic  AllPortsSameDT=off  OutDataTypeStr=boolean
  Logical Operator : Logic  Operator=NOT  AllPortsSameDT=off  OutDataTypeStr=boolean
  Logical Operator3 : Logic  Operator=NOT  AllPortsSameDT=off  OutDataTypeStr=boolean
  Merge : Merge  Inputs=3
  SOC_Equalization : PowerDistribution_SOC_equalization/SOC_Equalization
  multiple_packs : Subsystem
  only_one_Pack : Subsystem
  vector_PowerDistribution : Outport
  wires:
  SOC_Equalization/1 -> Merge/2
  Dynamic_power_distribution/1 -> Merge/3
  Merge/1 -> vector_PowerDistribution/1
  Logical Operator/1 -> Logical Operator2/2
  Choice_Algorithm/1(b_Strategy_SOC_Equalization) -> Logical Operator1/2, Logical Operator/1
  [n_Bat_type_ID_i_Bat2] -> Choice_Algorithm/5(n_Bat_type_ID_Bat2)
  [n_Bat_type_ID_i_Bat3] -> Choice_Algorithm/6(n_Bat_type_ID_Bat3)
  [n_Bat_type_ID_i_Bat1] -> Choice_Algorithm/4(n_Bat_type_ID_Bat1)
  [b_Bat_available_b_Bat3] -> Choice_Algorithm/3(b_Bat_available_b_Bat3)
  [b_Bat_available_b_Bat2] -> Choice_Algorithm/2(b_Bat_available_b_Bat2)
  [b_Bat_available_b_Bat1] -> Choice_Algorithm/1(b_Bat_available_b_Bat1)
  Bus Selector2/2 -> [n_Bat_type_ID_i_Bat3]  "<n_bat_type_ID_i>"
  Bus Selector1/2 -> [n_Bat_type_ID_i_Bat2]  "<n_bat_type_ID_i>"
  Bus Selector/2 -> [n_Bat_type_ID_i_Bat1]  "<n_bat_type_ID_i>"
  Bus Selector2/1 -> [b_Bat_available_b_Bat3]  "<b_Bat_available_b>"
  Bus Selector1/1 -> [b_Bat_available_b_Bat2]  "<b_Bat_available_b>"
  Bus Selector/1 -> [b_Bat_available_b_Bat1]  "<b_Bat_available_b>"
  SB_BMS_3/1 -> Bus Selector2/1, SOC_Equalization/3, Dynamic_power_distribution/3
  SB_BMS_2/1 -> Bus Selector1/1, SOC_Equalization/2, Dynamic_power_distribution/2
  SB_BMS_1/1 -> Bus Selector/1, SOC_Equalization/1, Dynamic_power_distribution/1
  Logical Operator1/1 -> ?
  [b_Bat_available_b_Bat1] -> multiple_packs/1(b_Bat_available_b_Bat1)
  [b_Bat_available_b_Bat2] -> multiple_packs/2(b_Bat_available_b_Bat2)
  [b_Bat_available_b_Bat3] -> multiple_packs/3(b_Bat_available_b_Bat3)
  Logical Operator2/1 -> ?
  multiple_packs/1(b_MultiplePacks) -> Logical Operator2/1, Logical Operator1/1, Logical Operator3/1
  only_one_Pack/1(vector_PowerDistribution) -> Merge/1
  Logical Operator3/1 -> only_one_Pack/Enable
  [b_Bat_available_b_Bat1] -> only_one_Pack/1(b_Bat_available_b_Bat1)
  [b_Bat_available_b_Bat2] -> only_one_Pack/2(b_Bat_available_b_Bat2)
  [b_Bat_available_b_Bat3] -> only_one_Pack/3(b_Bat_available_b_Bat3)
  Constant/1 -> SOC_Equalization/Enable

== system HVModAL_Fahrzeugmodell/Energy Manager (Emg)/Battery Control/Driving_Mode/Strategy_Maximiziation_Driving_Range1 ==
  note: Maximierung der Reichweite
      | = Minimierung elektrischer Verluste (ohm‘sch + Nebenaggregate)
      | 	V.a. interessant bei Topologie mit nur einem klimatisierten Pack
      | Z.B. Betrieb am oberen Temperaturmaximum der Zellen (höhere Alterung, aber geringerer Kühlbedarf)
  note: Pload:
      | positive: discharge
      | negative:charge
  note: Battery1: High Energy
      | Battery2: High Power
  SB_BMS_1 : Inport
  SB_BMS_2 : Inport  Port=2
  SB_BMS_3 : Inport  Port=3
  SB_DCDC_1 : Inport  Port=4
  SB_DCDC_2 : Inport  Port=5
  SB_DCDC_3 : Inport  Port=6
  Action Port : ActionPort
  Add1 : Sum  Inputs=+++
  Bus Selector2 : BusSelector  OutputSignals=P_DClink_W
  Bus Selector3 : BusSelector  OutputSignals=P_DClink_W
  Bus Selector4 : BusSelector  OutputSignals=P_DClink_W
  Minloss Strategy : Subsystem
  vector_PowerDistribution : Outport
  P_exchange_Master_Slave : Outport  Port=2
  wires:
  Minloss Strategy/2(P_exchange_Master_Slave) -> P_exchange_Master_Slave/1
  SB_BMS_2/1 -> Minloss Strategy/2(SB_BMS_2)
  Minloss Strategy/1(vector_PowerDistribution) -> vector_PowerDistribution/1
  Add1/1 -> Minloss Strategy/4(Pload)
  SB_BMS_3/1 -> Minloss Strategy/3(SB_BMS_3)
  SB_BMS_1/1 -> Minloss Strategy/1(SB_BMS_1)
  Bus Selector4/1 -> Add1/3  "<P_DClink_W>"
  Bus Selector3/1 -> Add1/2  "<P_DClink_W>"
  Bus Selector2/1 -> Add1/1  "<P_DClink_W>"
  SB_DCDC_3/1 -> Bus Selector4/1
  SB_DCDC_2/1 -> Bus Selector3/1
  SB_DCDC_1/1 -> Bus Selector2/1

== system HVModAL_Fahrzeugmodell/Energy Manager (Emg)/Battery Control/Driving_Mode/Strategy_Minimization_Current_Trip_Costs ==
  note: Minimierung der Kosten für Fahrt
      | - Minimierung der zyklischen Alterung (kalendarische Alterung vernachlässigbar während Fahrtdauer)
      | - Einflussfaktoren
      | 	Direkt: Strom, Zyklentiefe
      | 	Indirekt: Batterietemperatur
      | --> detaillierte Kenntnisse der jeweiligen Batterie notwendig
      | --> Batteriemanagement muss eingebunden werden, z.B. mit einer Leistungsanfrage-Kostenfunktion:
      | 	Energie-Manager: „Wie viel kostet Leistung X für X Sekunden?“
      | 	Bat1: „0,01 ct / kW / kWh @ 15kW“, Bat2: 0,02 ct / kW / kWh @ 10kW“….
      | 	Energiemanager muss Gesamtkostenminimum finden
  Action Port : ActionPort  ActionType=case
  Constant : Constant  Value=0.8
  Constant1 : Constant
  Constant2 : Constant  Value=0.3
  Mux : Mux  Inputs=3
  Subtract : Sum  Inputs=-+-
  abs2perc : Gain  Gain=100
  abs2perc1 : Gain  Gain=100
  abs2perc2 : Gain  Gain=100
  vector_PowerDistribution : Outport
  wires:
  Mux/1 -> vector_PowerDistribution/1
  abs2perc2/1 -> Mux/3  "PowerShare_Bat3"
  abs2perc/1 -> Mux/1  "PowerShare_Bat1"
  abs2perc1/1 -> Mux/2  "PowerShare_Bat2"
  Constant2/1 -> Subtract/3, abs2perc2/1
  Subtract/1 -> abs2perc1/1
  Constant1/1 -> Subtract/2
  Constant/1 -> abs2perc/1, Subtract/1

== system HVModAL_Fahrzeugmodell/Energy Manager (Emg)/Battery Control/Driving_Mode/Strategy_Minimization_LifeCycleCosts ==
  Action Port : ActionPort  ActionType=case
  Constant : Constant  Value=0.8
  Constant1 : Constant
  Constant2 : Constant  Value=0.3
  Mux : Mux  Inputs=3
  Subtract : Sum  Inputs=-+-
  abs2perc : Gain  Gain=100
  abs2perc1 : Gain  Gain=100
  abs2perc2 : Gain  Gain=100
  vector_PowerDistribution : Outport
  wires:
  Mux/1 -> vector_PowerDistribution/1
  abs2perc2/1 -> Mux/3  "PowerShare_Bat3"
  abs2perc/1 -> Mux/1  "PowerShare_Bat1"
  abs2perc1/1 -> Mux/2  "PowerShare_Bat2"
  Constant2/1 -> Subtract/3, abs2perc2/1
  Subtract/1 -> abs2perc1/1
  Constant1/1 -> Subtract/2
  Constant/1 -> abs2perc/1, Subtract/1

== system HVModAL_Fahrzeugmodell/HV-Batteries (Hvb)/Bat_1/BMS_Bat_/Temp Regulation ==
  note: ActiveCoolingSwitchOnTemperature
  note: @ Mitsubishi i-MiEV:
      | Active AirCooling at fastcharging with battery temperature above 30°C
      | Passive AirCooling only at battery temperature above 25°C
  note: ActiveCoolingSwitchOffTemperature
  note: ActiveHeatingSwitchOnTemperature
  note: ActiveHeatingSwitchOffTemperature
  note: 0: No cooling
      | 1: Active Aircooling
      | 2: Refrigerant Cooling
      | 3: Liquid Cooling
      | 4:Passive Aircooling
  T_max : Inport
  Fast charging on : Inport  Port=2
  Abs : Abs
  Active AirCooling : Constant
  Compare : simulink/Logic and Bit Operations/Compare To Constant  relop=>=  const=30  OutDataTypeStr=boolean
  Compare1 : simulink/Logic and Bit Operations/Compare To Constant  relop=<  const=0  OutDataTypeStr=boolean
  Cooling on : Constant  Value=4
  Gain : Gain  Gain=1/20
  Liquid Cooling : Constant  Value=3
  Logical Op1 : Logic  Operator=OR  AllPortsSameDT=off  OutDataTypeStr=boolean
  Logical Op2 : Logic  Operator=OR  AllPortsSameDT=off  OutDataTypeStr=boolean
  Logical Operator : Logic  AllPortsSameDT=off  OutDataTypeStr=boolean
  Logical Op : Logic  AllPortsSameDT=off  OutDataTypeStr=boolean
  RelOp1 : RelationalOperator  Operator===  OutDataTypeStr=boolean
  RelOp2 : RelationalOperator  Operator===  OutDataTypeStr=boolean
  Relay : Relay  OnSwitchValue=25  OffSwitchValue=20
  RellOp : RelationalOperator  Operator===  OutDataTypeStr=boolean
  Sum : Sum  Inputs=|+-
  T_desired : Constant  Value=20
  Terminator1 : Terminator
  Velocity Air [m/s] : Constant  Value=mask_v_Radial_Fan
  cooling system : Constant  Value=mask_cooling_method
  Compressor Power Factor : Outport
  Forced Air Cooling on : Outport  Port=2
  Forced Cooled Coolant Cooling on : Outport  Port=3
  Active Heating on : Outport  Port=4
  Velocity Air : Outport  Port=5
  wires:
  T_desired/1 -> Sum/1
  T_max/1 -> Compare/1, Compare1/1, Relay/1, Sum/2
  Fast charging on/1 -> Logical Operator/2
  Compare/1 -> Logical Operator/1
  Logical Operator/1 -> Terminator1/1
  Sum/1 -> Abs/1
  Abs/1 -> Gain/1
  Gain/1 -> Compressor Power Factor/1
  Cooling on/1 -> RellOp/2
  cooling system/1 -> RelOp1/1, RelOp2/1, RellOp/1
  RellOp/1 -> Logical Op2/1
  Relay/1 -> Logical Op/2
  Active AirCooling/1 -> RelOp1/2
  Liquid Cooling/1 -> RelOp2/2
  Logical Op/1 -> Forced Cooled Coolant Cooling on/1
  Compare1/1 -> Active Heating on/1
  RelOp1/1 -> Logical Op2/2, Logical Op1/1
  Velocity Air [m/s]/1 -> Velocity Air/1
  Logical Op2/1 -> Forced Air Cooling on/1
  RelOp2/1 -> Logical Op1/2
  Logical Op1/1 -> Logical Op/1

== system HVModAL_Fahrzeugmodell/HV-Batteries (Hvb)/Bat_1/Temp_model/ActiveAirCoolingCompressor ==
  note: 0: No cooling
      | 1: Active Aircooling
      | 2: Refrigerant Cooling
      | 3: Liquid Cooling
      | 4:Passive Aircooling
  ForcedAir Cooling on : Inport
  Forced Cooled Coolant Cooling on : Inport  Port=2
  Compressor Power Factor : Inport  Port=3
  Velocity Airstream : Inport  Port=4
  Active AirCooling : Constant
  Logical Op2 : Logic  AllPortsSameDT=off  OutDataTypeStr=boolean
  No convection : Constant  Value=0
  P_max LiquidCoolingSys : Constant  Value=mask_P_max_disch*0.02
  P_max_compr [W] : Gain  Gain=mask_P_max_disch*0.02
  RellOp : RelationalOperator  Operator===  OutDataTypeStr=boolean
  Switch : Switch  Criteria=u2 > Threshold  Threshold=1
  Switch1 : Switch  Criteria=u2 ~= 0  Threshold=1
  Switch3 : Switch  Criteria=u2 ~= 0  Threshold=1
  air_con_compr off : Constant  Value=0
  cooling system : Constant  Value=mask_cooling_method
  Velocity Air : Outport
  Q_dotActiveAirCooling : Outport  Port=2
  wires:
  air_con_compr off/1 -> Switch1/3
  Velocity Airstream/1 -> Switch3/1
  No convection/1 -> Switch3/3
  Switch3/1 -> Velocity Air/1
  Switch1/1 -> Q_dotActiveAirCooling/1
  ForcedAir Cooling on/1 -> Switch3/2
  P_max_compr [W]/1 -> Switch/3
  Compressor Power Factor/1 -> Switch/2, P_max_compr [W]/1
  Switch/1 -> Switch1/1
  P_max LiquidCoolingSys/1 -> Switch/1
  Forced Cooled Coolant Cooling on/1 -> Logical Op2/1
  RellOp/1 -> Logical Op2/2
  cooling system/1 -> RellOp/1
  Active AirCooling/1 -> RellOp/2
  Logical Op2/1 -> Switch1/2
